simulink model "SystemeCompletProcedural_original"  (R2019b)
settings: Solver=FixedStepAuto  StartTime=0  StopTime=5  FixedStep=0.0001  RelTol=1e-3
settings Model: Creator=jeanz  LastModifiedBy=maxim

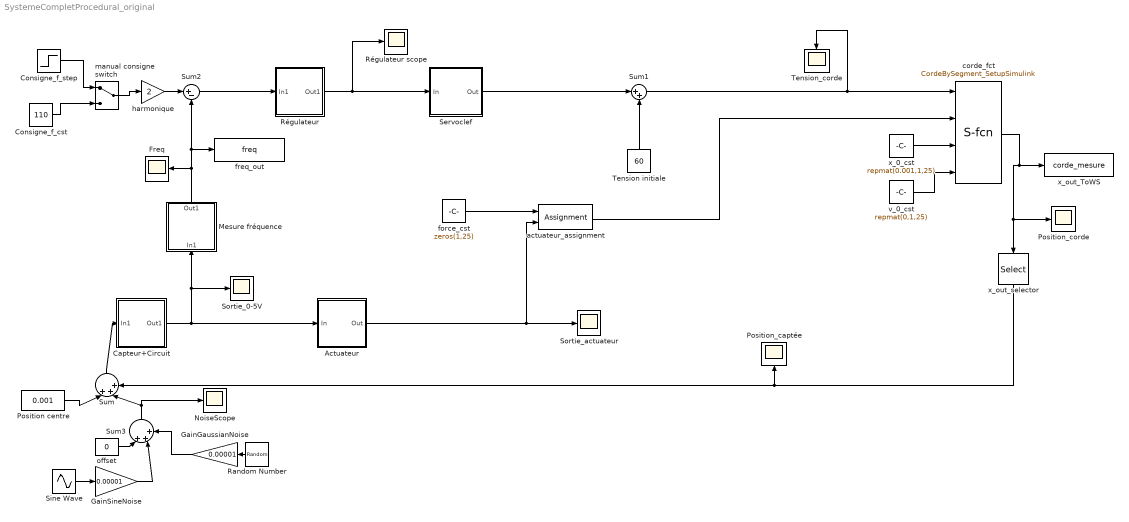
== system SystemeCompletProcedural_original ==
  Actuateur : Subsystem
  Capteur+Circuit : Subsystem
  Consigne_f_cst : Constant  Value=110
  Consigne_f_step : Step  Time=3  Before=80  After=120  SampleTime=0
  Freq : Scope
  GainGaussianNoise : Gain  Gain=0.00001
  GainSineNoise : Gain  Gain=0.00001
  Mesure fréquence : Subsystem
  NoiseScope : Scope
  Position centre : Constant  Value=0.001
  Position_captée : Scope
  Position_corde : Scope
  Random Number : RandomNumber  SampleTime=0.1
  Régulateur : Subsystem
  Régulateur scope : Scope
  Servoclef : Subsystem
  Sine Wave : Sin  SampleTime=0
  Sortie_0-5V : Scope
  Sortie_actuateur : Scope
  Sum : Sum  Inputs=|+++
  Sum1 : Sum  Inputs=|++
  Sum2 : Sum  Inputs=|+-
  Sum3 : Sum  Inputs=|+++
  Tension initiale : Constant  Value=60
  Tension_corde : Scope
  actuateur_assignment : Assignment  DiagnosticForDimensions=Warning  IndexOptions=Starting index (dialog)  Indices=20  OutputSizes=1
  corde_fct : M-S-Function  FunctionName=CordeBySegment_SetupSimulink  Parameters=3.250000e-03, 4.430000e-01, 3.260000e-02, 25, 1.000000e-04
  force_cst : Constant  Value=zeros(1,25)
  freq_out : ToWorkspace  VariableName=freq  SaveFormat=Timeseries  SampleTime=-1
  harmonique : Gain  Gain=2
  manual consigne switch : ManualSwitch
  offset : Constant  Value=0
  v_0_cst : Constant  Value=repmat(0,1,25)
  x_0_cst : Constant  Value=repmat(0.001,1,25)
  x_out_ToWS : ToWorkspace  VariableName=corde_mesure  SaveFormat=Timeseries  SampleTime=-1
  x_out_selector : Selector  IndexOptions=Starting index (dialog)  Indices=7  OutputSizes=1
  wires:
  actuateur_assignment/1 -> corde_fct/2
  corde_fct/1 -> x_out_ToWS/1, x_out_selector/1, Position_corde/1
  Capteur+Circuit/1(Out1) -> Sortie_0-5V/1, Mesure fréquence/1(In1), Actuateur/1(In)
  Mesure fréquence/1(Out1) -> Freq/1, Sum2/2, freq_out/1
  Sum/1 -> Capteur+Circuit/1(In1)
  Position centre/1 -> Sum/1
  Tension initiale/1 -> Sum1/2
  Servoclef/1(Out) -> Sum1/1
  Régulateur/1(Out1) -> Servoclef/1(In), Régulateur scope/1
  Sum2/1 -> Régulateur/1(In1)
  x_out_selector/1 -> Sum/3, Position_captée/1
  Sum1/1 -> Tension_corde/1, corde_fct/1
  x_0_cst/1 -> corde_fct/3
  v_0_cst/1 -> corde_fct/4
  Actuateur/1(Out) -> Sortie_actuateur/1, actuateur_assignment/2
  force_cst/1 -> actuateur_assignment/1
  harmonique/1 -> Sum2/1
  Consigne_f_cst/1 -> manual consigne switch/2
  manual consigne switch/1 -> harmonique/1
  Consigne_f_step/1 -> manual consigne switch/1
  Sine Wave/1 -> GainSineNoise/1
  Random Number/1 -> GainGaussianNoise/1
  GainSineNoise/1 -> Sum3/2
  GainGaussianNoise/1 -> Sum3/3
  offset/1 -> Sum3/1
  Sum3/1 -> NoiseScope/1, Sum/2

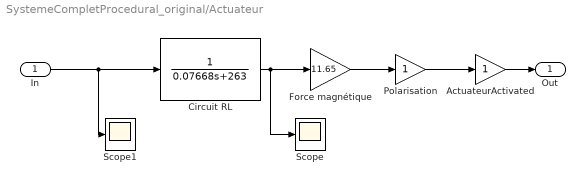
== system SystemeCompletProcedural_original/Actuateur ==
  In : Inport
  ActuateurActivated : Gain
  Circuit RL : TransferFcn  Denominator=[0.07668 263]
  Force magnétique : Gain  Gain=11.65
  Polarisation : Gain
  Scope : Scope
  Scope1 : Scope
  Out : Outport
  wires:
  Force magnétique/1 -> Polarisation/1
  Circuit RL/1 -> Force magnétique/1, Scope/1
  In/1 -> Scope1/1, Circuit RL/1
  Polarisation/1 -> ActuateurActivated/1
  ActuateurActivated/1 -> Out/1

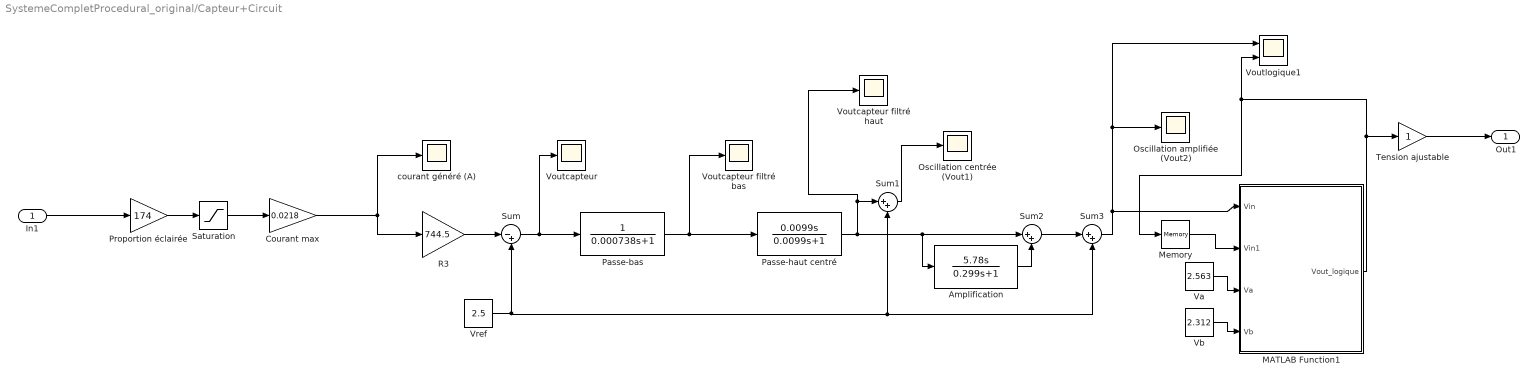
== system SystemeCompletProcedural_original/Capteur+Circuit ==
  In1 : Inport
  "Amplification " : TransferFcn  Numerator=[5.78 0]  Denominator=[0.299 1]
  Courant max : Gain  Gain=0.0218
  MATLAB Function1 : MATLAB Function  TreatAsAtomicUnit=on
  Memory : Memory
  "Oscillation amplifiée (Vout2) " : Scope
  Oscillation centrée (Vout1) : Scope
  Passe-bas : TransferFcn  Denominator=[0.000738 1]
  "Passe-haut centré " : TransferFcn  Numerator=[0.0099 0]  Denominator=[0.0099 1]
  Proportion éclairée : Gain  Gain=174
  R3 : Gain  Gain=744.5
  Saturation : Saturate  UpperLimit=0.497  LowerLimit=0
  Sum : Sum  Inputs=|-+
  Sum1 : Sum  Inputs=|++
  Sum2 : Sum  Inputs=|++
  Sum3 : Sum  Inputs=|++
  Tension ajustable : Gain
  "Va " : Constant  Value=2.563
  Vb : Constant  Value=2.312
  "Voutcapteur " : Scope
  Voutcapteur filtré bas : Scope
  Voutcapteur filtré haut : Scope
  Voutlogique1 : Scope  NumInputPorts=2
  "Vref " : Constant  Value=2.5
  "courant généré (A) " : Scope
  Out1 : Outport
  wires:
  Saturation/1 -> Courant max/1
  Tension ajustable/1 -> Out1/1
  Proportion éclairée/1 -> Saturation/1
  "Va "/1 -> MATLAB Function1/3(Va)
  Sum1/1 -> Oscillation centrée (Vout1)/1
  MATLAB Function1/1(Vout_logique) -> Memory/1, Voutlogique1/2, Tension ajustable/1
  "Vref "/1 -> Sum/2, Sum3/2, Sum1/2
  Sum2/1 -> Sum3/1
  Vb/1 -> MATLAB Function1/4(Vb)
  "Passe-haut centré "/1 -> Sum2/1, "Amplification "/1, Voutcapteur filtré haut/1, Sum1/1
  Memory/1 -> MATLAB Function1/2(Vin1)
  Sum/1 -> "Voutcapteur "/1, Passe-bas/1
  In1/1 -> Proportion éclairée/1
  Passe-bas/1 -> Voutcapteur filtré bas/1, "Passe-haut centré "/1
  Sum3/1 -> Voutlogique1/1, "Oscillation amplifiée (Vout2) "/1, MATLAB Function1/1(Vin)
  Courant max/1 -> R3/1, "courant généré (A) "/1
  "Amplification "/1 -> Sum2/2
  R3/1 -> Sum/1

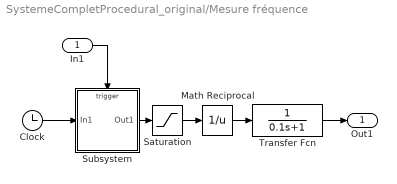
== system SystemeCompletProcedural_original/Mesure fréquence ==
  In1 : Inport
  Clock : Clock
  Math Reciprocal : Math  Operator=reciprocal  SaturateOnIntegerOverflow=on
  Saturation : Saturate  UpperLimit=1  LowerLimit=0.001
  Subsystem : Subsystem
  Transfer Fcn : TransferFcn  Denominator=[0.1 1]
  Out1 : Outport
  wires:
  In1/1 -> Subsystem/Trigger
  Clock/1 -> Subsystem/1(In1)
  Subsystem/1(Out1) -> Saturation/1
  Saturation/1 -> Math Reciprocal/1
  Math Reciprocal/1 -> Transfer Fcn/1
  Transfer Fcn/1 -> Out1/1

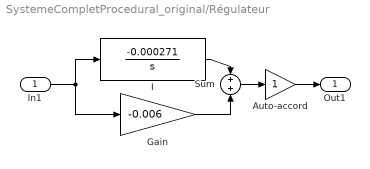
== system SystemeCompletProcedural_original/Régulateur ==
  In1 : Inport
  Auto-accord : Gain
  Gain : Gain  Gain=-0.006
  I : TransferFcn  Numerator=[-0.000271]  Denominator=[1 0]
  Sum : Sum  Inputs=+|+
  Out1 : Outport
  wires:
  In1/1 -> Gain/1, I/1
  Sum/1 -> Auto-accord/1
  I/1 -> Sum/1
  Gain/1 -> Sum/2
  Auto-accord/1 -> Out1/1

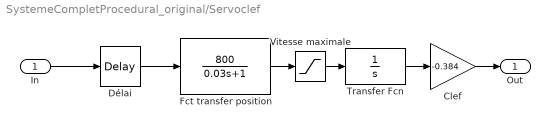
== system SystemeCompletProcedural_original/Servoclef ==
  In : Inport
  Clef : Gain  Gain=-0.384
  Délai : TransportDelay  DelayTime=0.01
  Fct transfer position : TransferFcn  Numerator=[800]  Denominator=[0.03 1]
  Transfer Fcn : TransferFcn  Denominator=[1 0]
  Vitesse maximale : Saturate  UpperLimit=1000  LowerLimit=-1000
  Out : Outport
  wires:
  Vitesse maximale/1 -> Transfer Fcn/1
  Fct transfer position/1 -> Vitesse maximale/1
  Clef/1 -> Out/1
  Délai/1 -> Fct transfer position/1
  In/1 -> Délai/1
  Transfer Fcn/1 -> Clef/1

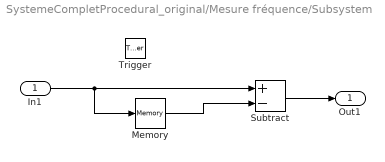
== system SystemeCompletProcedural_original/Mesure fréquence/Subsystem ==
  In1 : Inport
  Trigger : TriggerPort  VariantControl=Variant  PortDimensions=1
  Memory : Memory  InheritSampleTime=on
  Subtract : Sum  Inputs=+-
  Out1 : Outport
  wires:
  In1/1 -> Memory/1, Subtract/1
  Memory/1 -> Subtract/2
  Subtract/1 -> Out1/1

== matlab function SystemeCompletProcedural_original/Capteur+Circuit/MATLAB Function1 ==
  data: Vin input; Vin1 input; Vout_logique output; Va input; Vb input
function Vout_logique = fcn(Vin, Vin1 , Va, Vb)
Vout_logique = Vin1;
if Vin > Va && Vin1 == 5
    Vout_logique = 0;
end
if Vin < Vb && Vin1 == 0
    Vout_logique = 5;
end
end
